simulink model "bldc_DTC_final"  (R2024b)
settings: Solver=VariableStepAuto  StartTime=0.0  StopTime=13  RelTol=1e-3
model workspace (MAT data in the model file):
  Ls = 0.0027
  Rs = 0.7
libraries: spsIGBTDiodeLib x6, spsVoltageMeasurementLib x3, simulink x2, spsPermanentMagnetSynchronousMachineLib x1, spsDCVoltageSourceLib x1, simulink_extras x1, slpidlib x1, spsThreePhaseVIMeasurementLib x1, spspowerguiLib x1
settings Model: Creator=INNAGOL2  LastModifiedBy=INNAGOL2

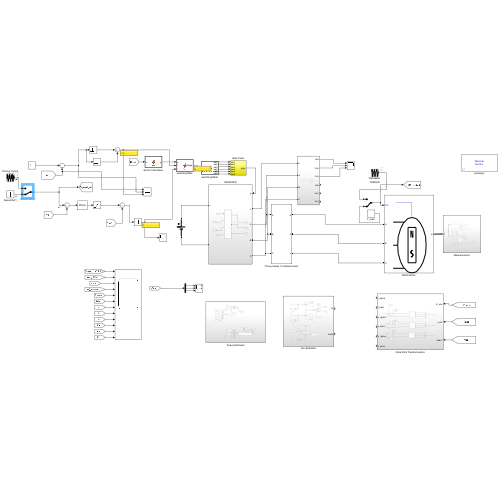
[thumbnail: Simulink's stored preview of the top-level diagram]
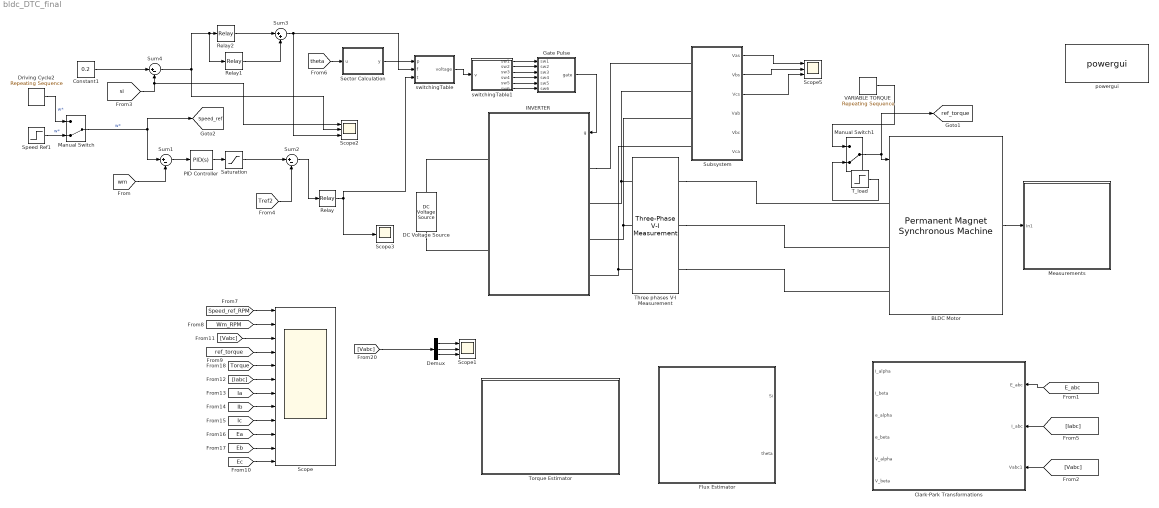
== system bldc_DTC_final ==
  BLDC Motor : spsPermanentMagnetSynchronousMachineLib/Permanent Magnet Synchronous Machine  NbPhases=3  FluxDistribution=Trapezoidal  RotorType=Round  MechanicalLoad=Torque Tm  PresetModel=No  ShowDetailedParameters=on  MeasurementBus=off  Resistance=0.7  Inductance=2.7e-3  dqInductances=[8.5e-3,8.5e-3]  La=0.000835  MachineConstant=Flux linkage established by magnets (V.s)  Flux=0.1194  VoltageCst=100.0283  TorqueCst=0.9552  Flat=120  Mechanical=[0.0027 0.0004924 4]  PolePairs=4  InitialConditions=[0,0, 0,0]  InitialConditions5ph=[0 0 0 0 0 0]  RefAngle=Aligned with phase A axis (original Park)  IterativeDiscreteModel=Trapezoidal non iterative  TsBlock=-1  TsPowergui=0
  Clark-Park Transformations : Subsystem
  Constant1 : Constant  Value=0.2
  DC Voltage Source : spsDCVoltageSourceLib/DC Voltage Source  Amplitude=160  Measurements=None
  Demux : Demux  Outputs=3
  Driving Cycle2 : simulink/Sources/Repeating Sequence  rep_seq_t=[0 1 2 3 4 5 6 7 8 9 10 11 11.0001 12 13]  rep_seq_y=[0 200 200 0 0 0 -100 -100 0 0 150 150 140 140 0]
  Flux Estimator : Subsystem
  Gate Pulse : Subsystem
  INVERTER : Subsystem
  Manual Switch : ManualSwitch  CurrentSetting=0
  Manual Switch1 : ManualSwitch  CurrentSetting=0
  Measurements : Subsystem
  PID Controller : slpidlib/PID Controller  Controller=PID  Form=Parallel  TimeDomain=Continuous-time  UseExternalTs=off  SampleTime=-1  IntegratorMethod=Forward Euler  FilterMethod=Forward Euler  ControllerParametersSource=internal  P=18  I=35  UseKiTs=off  D=0  UseExternalDerivativeSource=off  N=100  UseFilter=on  TunerSelectOption=Transfer Function Based (PID Tuner App)  InitialConditionSource=internal  InitialConditionForIntegrator=0  InitialConditionForFilter=0  DifferentiatorICPrevScaledInput=0  ExternalReset=none  TrackingMode=off  Kt=1  LimitOutput=off  SatLimitsSource=internal  UpperSaturationLimit=inf  LowerSaturationLimit=-inf  LinearizeAsGain=on  AntiWindupMode=none  Kb=1  LimitIntegrator=off  UpperIntegratorSaturationLimit=inf  LowerIntegratorSaturationLimit=-inf  POutMin=[]  POutMax=[]  IOutMin=[]  IOutMax=[]  DOutMin=[]  DOutMax=[]  NOutMin=[]  NOutMax=[]  SumOutMin=[]  SumOutMax=[]  SaturationOutMin=[]  SaturationOutMax=[]  PParamMin=[]  PParamMax=[]  IParamMin=[]  IParamMax=[]  DParamMin=[]  DParamMax=[]  NParamMin=[]  NParamMax=[]  KbParamMin=[]  KbParamMax=[]  KtParamMin=[]  KtParamMax=[]  KbOutMin=[]  KbOutMax=[]  KtOutMin=[]  KtOutMax=[]  IntegratorOutMin=[]  IntegratorOutMax=[]  FilterOutMin=[]  FilterOutMax=[]  SumI1OutMin=[]  SumI1OutMax=[]  SumI2OutMin=[]  SumI2OutMax=[]  SumI3OutMin=[]  SumI3OutMax=[]  SumI4OutMin=[]  SumI4OutMax=[]  SumDOutMin=[]  SumDOutMax=[]  DifferentiatorOutMin=[]  DifferentiatorOutMax=[]  FilterDiffOutCoefMin=[]  FilterDiffOutCoefMax=[]  ReciprocalOutMin=[]  ReciprocalOutMax=[]  SumDenOutMin=[]  SumDenOutMax=[]  SumNumOutMin=[]  SumNumOutMax=[]  DivideOutMin=[]  DivideOutMax=[]  UdiffTsProdOutMin=[]  UdiffTsProdOutMax=[]  NTsProdOutMin=[]  NTsProdOutMax=[]  UintegralTsProdOutMin=[]  UintegralTsProdOutMax=[]  UngainTsProdOutMin=[]  UngainTsProdOutMax=[]  ClampingZeroOutDataTypeStr=Inherit: Inherit via back propagation  ClampingZeroOutMin=[]  ClampingZeroOutMax=[]  FilterDenConstantOutDataTypeStr=Inherit: Inherit via back propagation  FilterDenConstantOutMin=[]  FilterDenConstantOutMax=[]  PCopyOutDataTypeStr=Inherit: Inherit via back propagation  PCopyOutMin=[]  PCopyOutMax=[]  NCopyOutDataTypeStr=Inherit: Inherit via back propagation  NCopyOutMin=[]  NCopyOutMax=[]  IntegratorContinuousStateAttributes=''  IntegratorStateMustResolveToSignalObject=off  IntegratorRTWStateStorageClass=Auto  FilterContinuousStateAttributes=''  FilterStateMustResolveToSignalObject=off  FilterRTWStateStorageClass=Auto  ParallelPVariant=InternalParameters  IdealPVariant=Disabled  IVariant=InternalParameters  DVariant=InternalParameters  IntegratorVariant=Continuous  SatVariant=Disabled  AWVariant=Passthrough  PCopyVariant=Disabled  TRVariant=Disabled  FdbkBlocksVariant=Forward  IdealPFdbkVariant=Disabled  SatFdbkVariant=Disabled  DerivativeFilterVariant=ContFilter  NVariant=InternalParameters  NCopyVariant=Disabled  FilterICVariant=InternalICsFilter  IntegratorICVariant=InternalICs  ExternalResetVariant=Disabled  TRSumVariant=Passthrough  SumFdbkVariant=Disabled  SumVariant=Sum_PID  TsampFilterVariant=InternalTs  TsampNgainVariant=Passthrough  TsampIntegralVariant=Disabled_SignalSpec  ExternalSaturationOutDataTypeStr=Inherit: Same as second input  DerivativeSourceVariant=ErrorSignal  PreIntVariant=InternalPreInt
  Relay : Relay  OnSwitchValue=1  OffSwitchValue=0  OnOutputValue=1  OffOutputValue=-1
  Relay1 : Relay  OnSwitchValue=0  OffSwitchValue=-0.01  OnOutputValue=0  OffOutputValue=-1
  Relay2 : Relay  OnSwitchValue=0.01  OffSwitchValue=0
  Saturation : Saturate  UpperLimit=25  LowerLimit=-25
  Scope : Scope  NumInputPorts=12
  Scope1 : Scope  NumInputPorts=3
  Scope2 : Scope  NumInputPorts=3
  Scope3 : Scope
  Scope5 : Scope  NumInputPorts=3
  Sector Calculation : MATLAB Function  TreatAsAtomicUnit=on
  Speed Ref1 : Step  Time=0.1  After=-150  SampleTime=0
  Subsystem : Subsystem
  Sum1 : Sum  Inputs=|+-
  Sum2 : Sum  Inputs=|+-
  Sum3 : Sum  Inputs=|++
  Sum4 : Sum  Inputs=|+-
  "T_load " : Step  Time=0.1  After=5  SampleTime=0
  Three phases V-I Measurement : spsThreePhaseVIMeasurementLib/Three-Phase V-I Measurement  VoltageMeasurement=phase-to-phase  SetLabelV=on  LabelV=Vabc  Vpu=off  VpuLL=off  CurrentMeasurement=yes  SetLabelI=on  LabelI=Iabc  Ipu=off  Pbase=100e6  Vbase=500e3  OutputType=Complex  PhasorSimulation=off  PSBequivalent=0
  Torque Estimator : Subsystem
  VARIABLE TORQUE : simulink/Sources/Repeating Sequence  rep_seq_t=[0 1 2 3 4 5 6 7 8 9 10 11 12 13]  rep_seq_y=[3 3 3 3 5 5 5 -2 -2 -2 1 1 1 1 ]
  powergui : spspowerguiLib/powergui  Priority=1  SimulationMode=Discrete  SampleTime=5e-05  frequency=60  Iterations=50  frequencyindice=0  Pbase=100e6  ErrMax=1e-4  UnitsV=kV  UnitsW=MW  buscounter=0  FunctionMessages=off  echomessages=off  EnableUseOfTLC=off  CurrentSourceSwitches=off  DisableSnubberDevices=off  DisableRonSwitches=off  DisableVfSwitches=off  DisplayEquations=off  AutomaticDiscreteSolvers=off  SolverType=Tustin/Backward Euler (TBE)  Interpol=off  ExternalGateDelay=off  methode=off  Ts=100  x0status=blocks  SPID=on  SwTol=0  HookPort=off  NonlinearTolerance=1e-4  nMaxIteration=100  ContinueOnMaxIteration=off  RestoreLinks=warning  ResistiveCurrentMeasurement=off  Frange=[0:2:500]  Ylog=off  Xlog=on  ShowGrid=off  save=off  variable=ZData  structure=0  ZoomFFT=off  StartTime=0.0  cycles=1  DisplayStyle=1  fundamental=60  FreqAxis=off  MaxFrequency=1000  frequencyindicesteady=1  RmsSteady=1  display=off
  switchingTable : MATLAB Function  TreatAsAtomicUnit=on
  switchingTable1 : MATLAB Function  TreatAsAtomicUnit=on
  tag scope: Speed_ref=global, ref_torque=global
  wires:
  PID Controller/1 -> Saturation/1
  Sum1/1 -> PID Controller/1
  Constant1/1 -> Sum4/1
  [wm] -> Sum1/2
  Saturation/1 -> Sum2/1
  VARIABLE TORQUE/1 -> Manual Switch1/1
  Manual Switch1/1 -> BLDC Motor/1, [ref_torque]
  Gate Pulse/1(gate) -> INVERTER/1(g)
  BLDC Motor/1 -> Measurements/1(In1)
  "T_load "/1 -> Manual Switch1/2
  [Iabc] -> Clark-Park Transformations/2(I_abc)
  [E_abc] -> Clark-Park Transformations/1(E_abc)
  [Vabc] -> Clark-Park Transformations/3(Vabc1)
  Manual Switch/1 -> Sum1/1, [Speed_ref]  "w*"
  Sum2/1 -> Relay/1
  Sum4/1 -> Scope2/2, Relay1/1, Relay2/1
  [si] -> Scope2/1, Sum4/2
  [Tref2] -> Sum2/2
  Sector Calculation/1(y) -> switchingTable/1(p)
  [theta] -> Sector Calculation/1(u)
  [Ic] -> Scope/9
  [Ec] -> Scope/12
  [Ea] -> Scope/10
  [Eb] -> Scope/11
  [Vabc] -> Scope/3
  [Torque] -> Scope/5
  [Wm_RPM] -> Scope/2
  [Iabc] -> Scope/6
  [Ib] -> Scope/8
  [Ia] -> Scope/7
  [ref_torque] -> Scope/4
  [Speed_ref_RPM] -> Scope/1
  Driving Cycle2/1 -> Manual Switch/1  "w*"
  Speed Ref1/1 -> Manual Switch/2  "w*"
  [Vabc] -> Demux/1
  Demux/1 -> Scope1/1
  Demux/2 -> Scope1/2
  Demux/3 -> Scope1/3
  Relay/1 -> Scope3/1, switchingTable/3(t)
  switchingTable1/1(sw1) -> Gate Pulse/1(sw1)
  switchingTable1/2(sw2) -> Gate Pulse/2(sw2)
  switchingTable1/3(sw3) -> Gate Pulse/3(sw3)
  switchingTable1/4(sw4) -> Gate Pulse/4(sw4)
  switchingTable1/5(sw5) -> Gate Pulse/5(sw5)
  switchingTable1/6(sw6) -> Gate Pulse/6(sw6)
  switchingTable/1(voltage) -> switchingTable1/1(v)
  Relay2/1 -> Sum3/1
  Relay1/1 -> Sum3/2
  Sum3/1 -> Scope2/3, switchingTable/2(f)
  Subsystem/1(Vas) -> Scope5/1
  Subsystem/2(Vbs) -> Scope5/2
  Subsystem/3(Vcs) -> Scope5/3
  connections:
  Three phases V-I Measurement/LConn3 -- Subsystem/LConn4 -- INVERTER/LConn4
  DC Voltage Source/RConn1 -- INVERTER/RConn1
  Three phases V-I Measurement/LConn2 -- INVERTER/LConn3 -- Subsystem/LConn3
  DC Voltage Source/LConn1 -- INVERTER/RConn2
  Three phases V-I Measurement/LConn1 -- Subsystem/LConn2 -- INVERTER/LConn2
  INVERTER/LConn1 -- Subsystem/LConn1
  Three phases V-I Measurement/RConn1 -- BLDC Motor/LConn1
  Three phases V-I Measurement/RConn2 -- BLDC Motor/LConn2
  Three phases V-I Measurement/RConn3 -- BLDC Motor/LConn3

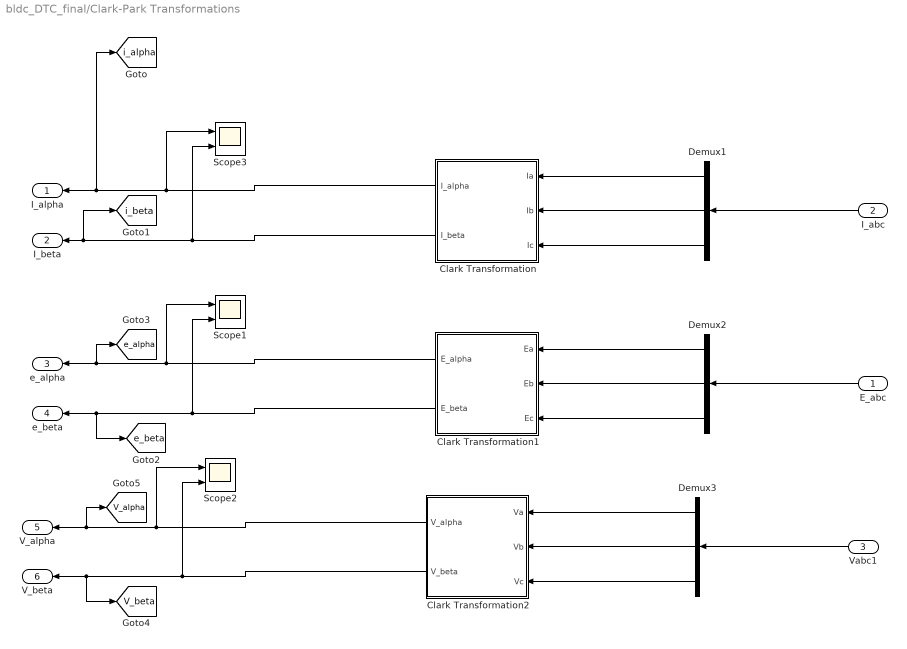
== system bldc_DTC_final/Clark-Park Transformations ==
  E_abc : Inport
  I_abc : Inport  Port=2
  Vabc1 : Inport  Port=3
  Clark Transformation : Subsystem
  Clark Transformation1 : Subsystem
  Clark Transformation2 : Subsystem
  Demux1 : Demux  Outputs=3
  Demux2 : Demux  Outputs=3
  Demux3 : Demux  Outputs=3
  Scope1 : Scope  NumInputPorts=2
  Scope2 : Scope  NumInputPorts=2
  Scope3 : Scope  NumInputPorts=2
  I_alpha : Outport
  I_beta : Outport  Port=2
  e_alpha : Outport  Port=3
  e_beta : Outport  Port=4
  V_alpha : Outport  Port=5
  V_beta : Outport  Port=6
  tag scope: V_alpha=global, V_beta=global, e_alpha=global, e_beta=global, i_alpha=global, i_beta=global
  wires:
  Demux1/1 -> Clark Transformation/1(Ia)
  Demux1/2 -> Clark Transformation/2(Ib)
  Demux1/3 -> Clark Transformation/3(Ic)
  I_abc/1 -> Demux1/1
  Clark Transformation/1(I_alpha) -> Scope3/1, [i_alpha], I_alpha/1
  Clark Transformation/2(I_beta) -> Scope3/2, [i_beta], I_beta/1
  Clark Transformation1/2(E_beta) -> [e_beta], e_beta/1, Scope1/2
  Clark Transformation1/1(E_alpha) -> [e_alpha], e_alpha/1, Scope1/1
  E_abc/1 -> Demux2/1
  Demux2/3 -> Clark Transformation1/3(Ec)
  Demux2/2 -> Clark Transformation1/2(Eb)
  Demux2/1 -> Clark Transformation1/1(Ea)
  Demux3/1 -> Clark Transformation2/1(Va)
  Demux3/2 -> Clark Transformation2/2(Vb)
  Demux3/3 -> Clark Transformation2/3(Vc)
  Vabc1/1 -> Demux3/1
  Clark Transformation2/1(V_alpha) -> Scope2/1, V_alpha/1, [V_alpha]
  Clark Transformation2/2(V_beta) -> Scope2/2, V_beta/1, [V_beta]

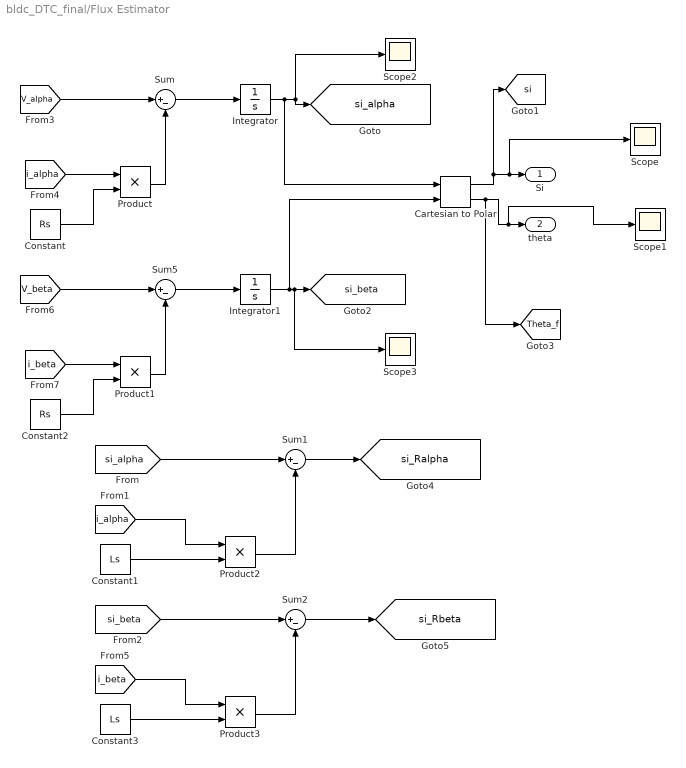
== system bldc_DTC_final/Flux Estimator ==
  Cartesian to Polar : simulink_extras/Transformations/Cartesian to Polar
  Constant : Constant  Value=Rs
  Constant1 : Constant  Value=Ls
  Constant2 : Constant  Value=Rs
  Constant3 : Constant  Value=Ls
  Integrator : Integrator
  Integrator1 : Integrator
  Product{,1..3} (4 alike) : Product
  Scope{,1..3} (4 alike) : Scope
  Sum{,1..2,5} (4 alike) : Sum  Inputs=|+-
  Si : Outport
  theta : Outport  Port=2
  tag scope: Theta_f=global, si=global, si_Ralpha=global, si_Rbeta=global, si_alpha=global, si_beta=global
  wires:
  Constant/1 -> Product/2
  Integrator/1 -> Cartesian to Polar/1, Scope2/1, [si_alpha]
  [V_alpha] -> Sum/1
  [i_alpha] -> Product/1
  Product1/1 -> Sum5/2
  Product/1 -> Sum/2
  [i_beta] -> Product1/1
  Constant2/1 -> Product1/2
  Sum5/1 -> Integrator1/1
  [V_beta] -> Sum5/1
  Integrator1/1 -> Cartesian to Polar/2, Scope3/1, [si_beta]
  Sum/1 -> Integrator/1
  Cartesian to Polar/1 -> [si], Scope/1, Si/1
  Cartesian to Polar/2 -> [Theta_f], Scope1/1, theta/1
  [si_alpha] -> Sum1/1
  [i_alpha] -> Product2/1
  Constant1/1 -> Product2/2
  Product2/1 -> Sum1/2
  Product3/1 -> Sum2/2
  Constant3/1 -> Product3/2
  [i_beta] -> Product3/1
  [si_beta] -> Sum2/1
  Sum1/1 -> [si_Ralpha]
  Sum2/1 -> [si_Rbeta]

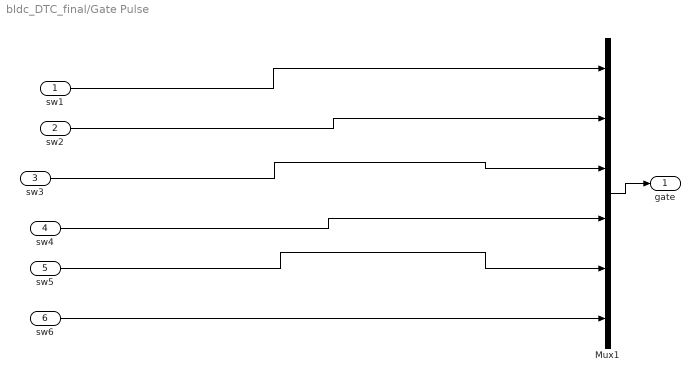
== system bldc_DTC_final/Gate Pulse ==
  sw1 : Inport
  sw2 : Inport  Port=2
  sw3 : Inport  Port=3
  sw4 : Inport  Port=4
  sw5 : Inport  Port=5
  sw6 : Inport  Port=6
  Mux1 : Mux  Inputs=6
  gate : Outport
  wires:
  sw5/1 -> Mux1/5
  Mux1/1 -> gate/1
  sw3/1 -> Mux1/3
  sw1/1 -> Mux1/1
  sw2/1 -> Mux1/2
  sw4/1 -> Mux1/4
  sw6/1 -> Mux1/6

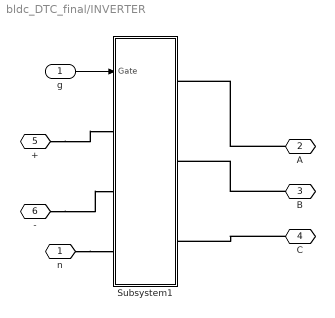
== system bldc_DTC_final/INVERTER ==
  g : Inport
  Subsystem1 : Subsystem
  " n" : PMIOPort  Side=Left
  A : PMIOPort  Port=2  Side=Left
  B : PMIOPort  Port=3  Side=Left
  C : PMIOPort  Port=4  Side=Left
  + : PMIOPort  Port=5  Side=Right
  - : PMIOPort  Port=6  Side=Right
  wires:
  g/1 -> Subsystem1/1(Gate)
  connections:
  +/RConn1 -- Subsystem1/LConn1
  -/RConn1 -- Subsystem1/LConn2
  C/RConn1 -- Subsystem1/RConn3
  B/RConn1 -- Subsystem1/RConn2
  A/RConn1 -- Subsystem1/RConn1
  " n"/RConn1 -- Subsystem1/LConn3

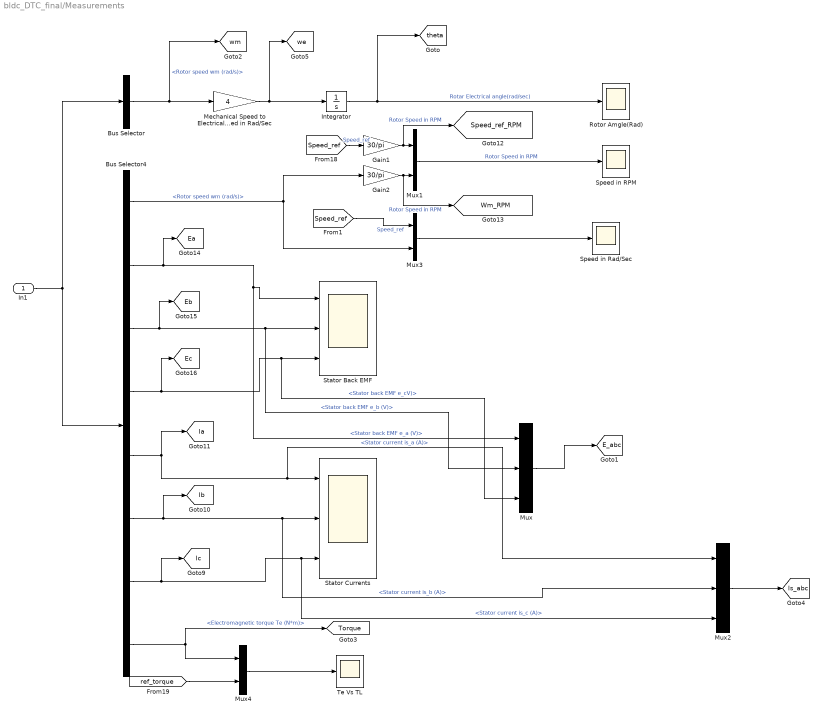
== system bldc_DTC_final/Measurements ==
  In1 : Inport
  Bus Selector : BusSelector  OutputSignals=Rotor speed wm (rad/s)
  Bus Selector4 : BusSelector  OutputSignals=Rotor speed wm (rad/s),Stator back EMF e_a (V),Stator back EMF e_b (V),Stator back EMF e_cV),Stator current is_a (A),Stator current is_b (A),Stator current is_c (A),Electromagnetic torque Te (N*m)
  Gain1 : Gain  Gain=30/pi
  Gain2 : Gain  Gain=30/pi
  Integrator : Integrator  WrapState=on
  Mechanical Speed to Electrical speed in Rad/Sec : Gain  Gain=4
  Mux : Mux  Inputs=3
  Mux1 : Mux  Inputs=2
  Mux2 : Mux  Inputs=3
  Mux3 : Mux  Inputs=2
  Mux4 : Mux  Inputs=2
  Rotor Amgle(Rad) : Scope
  Speed in RPM : Scope
  Speed in Rad/Sec : Scope
  Stator Back EMF : Scope  NumInputPorts=3
  Stator Currents : Scope  NumInputPorts=3
  Te Vs TL : Scope
  tag scope: E_abc=global, Ea=global, Eb=global, Ec=global, Ia=global, Ib=global, Ic=global, Is_abc=global, Speed_ref_RPM=global, Torque=global, Wm_RPM=global, theta=global, we=global, wm=global
  wires:
  [ref_torque] -> Mux4/2
  Mechanical Speed to Electrical speed in Rad/Sec/1 -> [we], Integrator/1
  Mux4/1 -> Te Vs TL/1
  Bus Selector/1 -> [wm], Mechanical Speed to Electrical speed in Rad/Sec/1  "<Rotor speed wm (rad/s)>"
  Bus Selector4/3 -> [Eb], Mux/2, Stator Back EMF/2  "<Stator back EMF e_b (V)>"
  Bus Selector4/8 -> [Torque], Mux4/1  "<Electromagnetic torque Te (N*m)>"
  Bus Selector4/5 -> [Ia], Mux2/1, Stator Currents/1  "<Stator current is_a (A)>"
  In1/1 -> Bus Selector4/1, Bus Selector/1
  Bus Selector4/4 -> [Ec], Mux/3, Stator Back EMF/3  "<Stator back EMF e_cV)>"
  Gain2/1 -> [Wm_RPM], Mux1/2  "Rotor Speed in RPM"
  Bus Selector4/7 -> [Ic], Mux2/3, Stator Currents/3  "<Stator current is_c (A)>"
  Integrator/1 -> [theta], Rotor Amgle(Rad)/1  "Rotar Electrical angle(rad/sec)"
  Bus Selector4/2 -> [Ea], Mux/1, Stator Back EMF/1  "<Stator back EMF e_a (V)>"
  Bus Selector4/1 -> Mux3/2, Gain2/1  "<Rotor speed wm (rad/s)>"
  Gain1/1 -> [Speed_ref_RPM], Mux1/1  "Rotor Speed in RPM"
  Mux3/1 -> Speed in Rad/Sec/1
  Mux1/1 -> Speed in RPM/1  "Rotor Speed in RPM"
  [Speed_ref] -> Gain1/1  "Speed_ref"
  Bus Selector4/6 -> [Ib], Mux2/2, Stator Currents/2  "<Stator current is_b (A)>"
  [Speed_ref] -> Mux3/1  "Speed_ref"
  Mux/1 -> [E_abc]
  Mux2/1 -> [Is_abc]

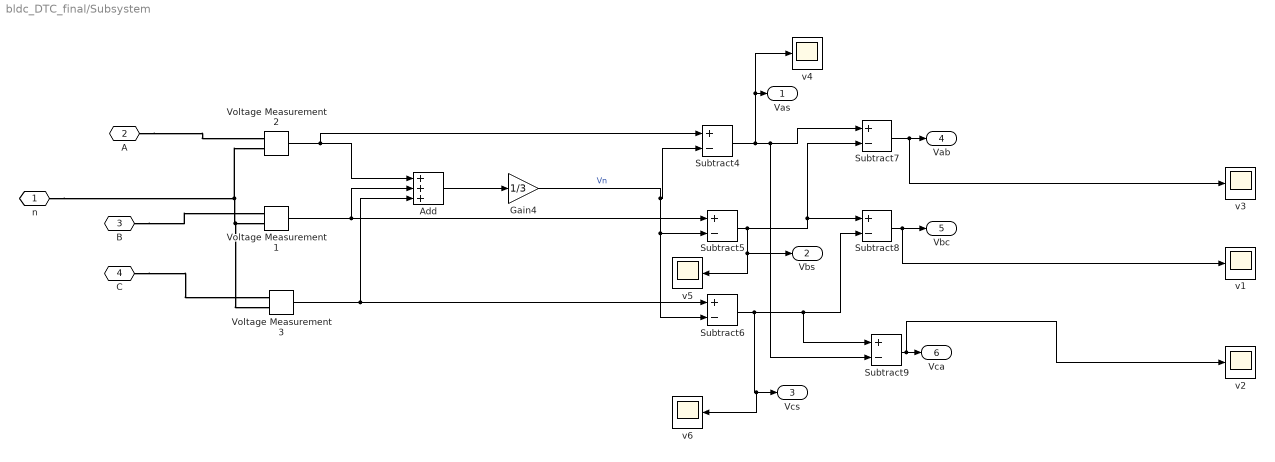
== system bldc_DTC_final/Subsystem ==
  Add : Sum  Inputs=+++
  Gain4 : Gain  Gain=1/3
  Subtract{4..9} (6 alike) : Sum  Inputs=+-
  Voltage Measurement1 : spsVoltageMeasurementLib/Voltage Measurement  PhasorSimulation=off  OutputType=Complex  PSBequivalent=0
  Voltage Measurement2 : spsVoltageMeasurementLib/Voltage Measurement  PhasorSimulation=off  OutputType=Complex  PSBequivalent=0
  Voltage Measurement3 : spsVoltageMeasurementLib/Voltage Measurement  PhasorSimulation=off  OutputType=Complex  PSBequivalent=0
  v{1..6} (6 alike) : Scope
  n : PMIOPort  Side=Left
  A : PMIOPort  Port=2  Side=Left
  B : PMIOPort  Port=3  Side=Left
  C : PMIOPort  Port=4  Side=Left
  Vas : Outport  VectorParamsAs1DForOutWhenUnconnected=off
  Vbs : Outport  Port=2  VectorParamsAs1DForOutWhenUnconnected=off
  Vcs : Outport  Port=3  VectorParamsAs1DForOutWhenUnconnected=off
  Vab : Outport  Port=4  VectorParamsAs1DForOutWhenUnconnected=off
  Vbc : Outport  Port=5  VectorParamsAs1DForOutWhenUnconnected=off
  Vca : Outport  Port=6  VectorParamsAs1DForOutWhenUnconnected=off
  wires:
  Voltage Measurement2/1 -> Subtract4/1, Add/1
  Voltage Measurement1/1 -> Subtract5/1, Add/2
  Voltage Measurement3/1 -> Subtract6/1, Add/3
  Add/1 -> Gain4/1
  Subtract4/1 -> v4/1, Vas/1, Subtract9/2, Subtract7/1
  Subtract5/1 -> v5/1, Vbs/1, Subtract8/1, Subtract7/2
  Subtract6/1 -> v6/1, Vcs/1, Subtract9/1, Subtract8/2
  Subtract7/1 -> v3/1, Vab/1
  Subtract8/1 -> v1/1, Vbc/1
  Subtract9/1 -> v2/1, Vca/1
  Gain4/1 -> Subtract6/2, Subtract5/2, Subtract4/2  "Vn"
  connections:
  n/RConn1 -- Voltage Measurement2/LConn2 -- Voltage Measurement3/LConn2 -- Voltage Measurement1/LConn2
  A/RConn1 -- Voltage Measurement2/LConn1
  B/RConn1 -- Voltage Measurement1/LConn1
  C/RConn1 -- Voltage Measurement3/LConn1

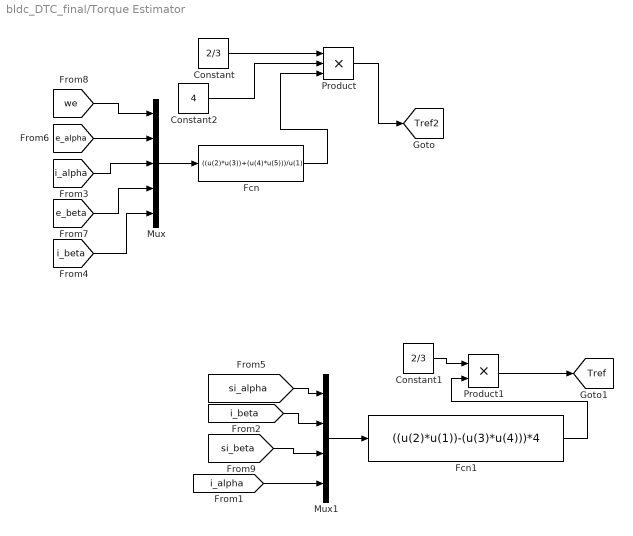
== system bldc_DTC_final/Torque Estimator ==
  Constant : Constant  Value=2/3
  Constant1 : Constant  Value=2/3
  Constant2 : Constant  Value=4
  Fcn : Fcn  Expr=((u(2)*u(3))+(u(4)*u(5)))/u(1)
  Fcn1 : Fcn  Expr=((u(2)*u(1))-(u(3)*u(4)))*4
  Mux : Mux  Inputs=5
  Mux1 : Mux
  Product : Product  Inputs=3
  Product1 : Product
  tag scope: Tref2=global, Tref=global
  wires:
  Constant/1 -> Product/1
  [i_beta] -> Mux/5
  [i_alpha] -> Mux/3
  Mux/1 -> Fcn/1
  Product/1 -> [Tref2]
  [e_beta] -> Mux/4
  Fcn/1 -> Product/3
  [we] -> Mux/1
  [e_alpha] -> Mux/2
  Constant2/1 -> Product/2
  [si_beta] -> Mux1/3
  [si_alpha] -> Mux1/1
  Mux1/1 -> Fcn1/1
  [i_beta] -> Mux1/2
  [i_alpha] -> Mux1/4
  Product1/1 -> [Tref]
  Constant1/1 -> Product1/1
  Fcn1/1 -> Product1/2

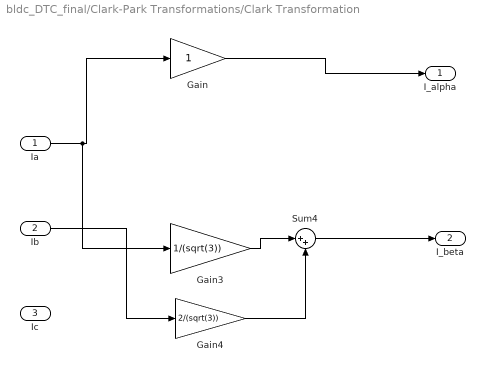
== system bldc_DTC_final/Clark-Park Transformations/Clark Transformation ==
  Ia : Inport
  Ib : Inport  Port=2
  Ic : Inport  Port=3
  Gain : Gain
  Gain3 : Gain  Gain=1/(sqrt(3))
  Gain4 : Gain  Gain=2/(sqrt(3))
  Sum4 : Sum  Inputs=|++
  I_alpha : Outport
  I_beta : Outport  Port=2
  wires:
  Gain/1 -> I_alpha/1
  Gain3/1 -> Sum4/1
  Gain4/1 -> Sum4/2
  Ia/1 -> Gain3/1, Gain/1
  Sum4/1 -> I_beta/1
  Ib/1 -> Gain4/1

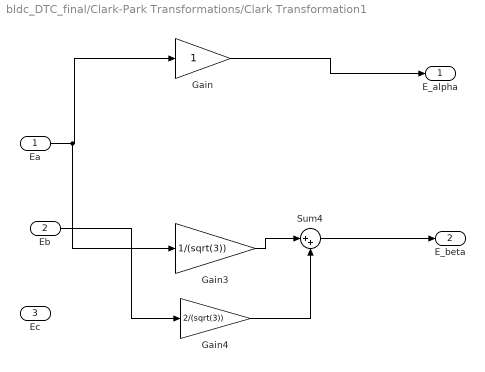
== system bldc_DTC_final/Clark-Park Transformations/Clark Transformation1 ==
  Ea : Inport
  Eb : Inport  Port=2
  Ec : Inport  Port=3
  Gain : Gain
  Gain3 : Gain  Gain=1/(sqrt(3))
  Gain4 : Gain  Gain=2/(sqrt(3))
  Sum4 : Sum  Inputs=|++
  E_alpha : Outport
  E_beta : Outport  Port=2
  wires:
  Gain/1 -> E_alpha/1
  Ea/1 -> Gain3/1, Gain/1
  Eb/1 -> Gain4/1
  Gain3/1 -> Sum4/1
  Sum4/1 -> E_beta/1
  Gain4/1 -> Sum4/2

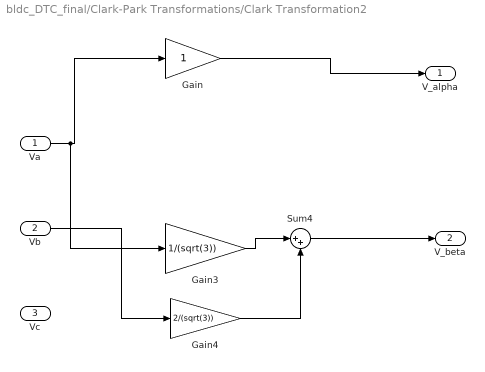
== system bldc_DTC_final/Clark-Park Transformations/Clark Transformation2 ==
  Va : Inport
  Vb : Inport  Port=2
  Vc : Inport  Port=3
  Gain : Gain
  Gain3 : Gain  Gain=1/(sqrt(3))
  Gain4 : Gain  Gain=2/(sqrt(3))
  Sum4 : Sum  Inputs=|++
  V_alpha : Outport
  V_beta : Outport  Port=2
  wires:
  Gain/1 -> V_alpha/1
  Va/1 -> Gain3/1, Gain/1
  Vb/1 -> Gain4/1
  Gain3/1 -> Sum4/1
  Sum4/1 -> V_beta/1
  Gain4/1 -> Sum4/2

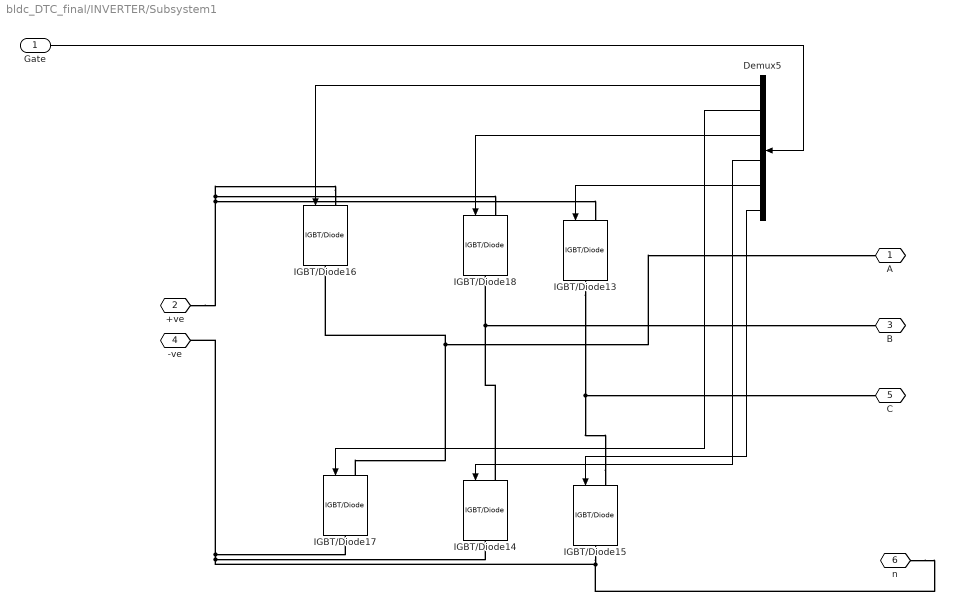
== system bldc_DTC_final/INVERTER/Subsystem1 ==
  Gate : Inport
  Demux5 : Demux  Outputs=6
  IGBT/Diode{13..18} (6 alike) : spsIGBTDiodeLib/IGBT//Diode  Ron=1e-3  Rs=1e5  Cs=inf  Measurements=off
  A : PMIOPort  Side=Right
  +ve : PMIOPort  Port=2  Side=Left
  B : PMIOPort  Port=3  Side=Right
  -ve : PMIOPort  Port=4  Side=Left
  C : PMIOPort  Port=5  Side=Right
  " n" : PMIOPort  Port=6  Side=Left
  wires:
  Gate/1 -> Demux5/1
  Demux5/1 -> IGBT/Diode16/1
  Demux5/2 -> IGBT/Diode17/1
  Demux5/3 -> IGBT/Diode18/1
  Demux5/4 -> IGBT/Diode14/1
  Demux5/5 -> IGBT/Diode13/1
  Demux5/6 -> IGBT/Diode15/1
  connections:
  IGBT/Diode15/LConn1 -- C/RConn1 -- IGBT/Diode13/RConn1
  IGBT/Diode18/RConn1 -- B/RConn1 -- IGBT/Diode14/LConn1
  IGBT/Diode14/RConn1 -- " n"/RConn1 -- IGBT/Diode15/RConn1 -- IGBT/Diode17/RConn1 -- -ve/RConn1
  IGBT/Diode16/RConn1 -- A/RConn1 -- IGBT/Diode17/LConn1
  IGBT/Diode16/LConn1 -- IGBT/Diode18/LConn1 -- +ve/RConn1 -- IGBT/Diode13/LConn1

== matlab function bldc_DTC_final/switchingTable ==
  data: p input; voltage output; f input; t input
function voltage = fcn(p, f, t)
    % Ensure inputs are doubles
    p = double(p);
    f = double(f);
    t = double(t);
    
    % Define the output as a scalar
    voltage = 0; % default value

    % Check if the inputs are valid (scalars)
    if numel(p) ~= 1 || numel(f) ~= 1 || numel(t) ~= 1
        error('Inputs p, f, and t must be scalars');
    end
    
    % Define the logic based on the voltage value of p
    if p == 1
        if f == 1 && t == 1
            voltage = 1;
        elseif f == 0 && t == 1
            voltage = 2;    
        elseif f == -1 && t == 1
            voltage = 3;
        elseif f == 1 && t == 0
            voltage = 1;
        elseif f == 0 && t == 0
            voltage = 0;   
        elseif f == -1 && t == 0
            voltage = 3;
        elseif f == 1 && t == -1
            voltage = 6;
        elseif f == 0 && t == -1
            voltage = 5;   
        elseif f == -1 && t == -1
            voltage = 4;
        end
    elseif p == 2
        if f == 1 && t == 1
            voltage = 2;
        elseif f == 0 && t == 1
            voltage = 3;    
        elseif f == -1 && t == 1
            voltage = 4;
         elseif f == 1 && t == 0
            voltage = 2;
        elseif f == 0 && t == 0
            voltage = 0;   
        elseif f == -1 && t == 0
            voltage = 4;
         elseif f == 1 && t == -1
            voltage = 1;
        elseif f == 0 && t == -1
            voltage = 6;   
        elseif f == -1 && t == -1
            voltage = 5;
        end
    elseif p == 3
        if f == 1 && t == 1
            voltage = 3;
        elseif f == 0 && t == 1
            voltage = 4;    
        elseif f == -1 && t == 1
            voltage = 5;
        elseif f == 1 && t == 0
            voltage = 3;
        elseif f == 0 && t == 0
            voltage = 0;   
        elseif f == -1 && t == 0
            voltage = 5;
        elseif f == 1 && t == -1
            voltage = 2;
        elseif f == 0 && t == -1
            voltage = 1;   
        elseif f == -1 && t == -1
            voltage = 6;        
        end
    elseif p == 4
        if f == 1 && t == 1
            voltage = 4;
        elseif f == 0 && t == 1
            voltage = 5;    
        elseif f == -1 && t == 1
            voltage = 6;
        elseif f == 1 && t == 0
            voltage = 4;
        elseif f == 0 && t == 0
            voltage = 0;   
        elseif f == -1 && t == 0
            voltage = 6;
        elseif f == 1 && t == -1
            voltage = 3;
        elseif f == 0 && t == -1
            voltage = 2;   
        elseif f == -1 && t == -1
            voltage = 1;
        end
    elseif p == 5
        if f == 1 && t == 1
            voltage = 5;
        elseif f == 0 && t == 1
            voltage = 6;    
        elseif f == -1 && t == 1
            voltage = 1;
        elseif f == 1 && t == 0
            voltage = 5;
        elseif f == 0 && t == 0
            voltage = 0;   
        elseif f == -1 && t == 0
            voltage = 1;
        elseif f == 1 && t == -1
            voltage = 4;
        elseif f == 0 && t == -1
            voltage = 3;   
        elseif f == -1 && t == -1
            voltage = 2;
        end
    elseif p == 6
        if f == 1 && t == 1
            voltage = 6;
        elseif f == 0 && t == 1
            voltage = 1;    
        elseif f == -1 && t == 1
            voltage = 2;
        elseif f == 1 && t == 0
            voltage = 6;
        elseif f == 0 && t == 0
            voltage = 0;   
        elseif f == -1 && t == 0
            voltage = 2;
        elseif f == 1 && t == -1
            voltage = 5;
        elseif f == 0 && t == -1
            voltage = 4;   
        elseif f == -1 && t == -1
            voltage = 3;
        end
    end
end

== matlab function bldc_DTC_final/Sector Calculation ==
  data: u input; y output
function y = fcn(u)
if ( u >- pi/6 && u<=pi / 6 )
y = 1;
elseif ( u > pi/6 && u <= pi / 2)
y = 2;
elseif (u > pi/2 && u<= 5*(pi/6))
y = 3;
elseif (u > - 5*(pi/6) && u<= -pi/2)
y = 5;
elseif ( u > - pi/2 && u<=-pi/6)
y = 6;
else
y = 4;
end

== matlab function bldc_DTC_final/switchingTable1 ==
  data: v input; sw1 output; sw2 output; sw3 output; sw4 output; sw5 output; sw6 output
function [sw1, sw2, sw3, sw4, sw5, sw6] = voltage_vector(v)
    % Initialize all switch outputs to 0
    sw1 = 0; sw2 = 0; sw3 = 0; sw4 = 0; sw5 = 0; sw6 = 0;
 
    % Determine the output based on inputs
    
            if v == 1
                sw1 = 1; sw2 = 0; sw3 = 0; sw4 = 0; sw5 = 0; sw6 = 1;
            elseif v == 2
                sw1 = 0; sw2 = 0; sw3 = 1; sw4 = 0; sw5 = 0; sw6 = 1;
            elseif v == 3
                sw1 = 0; sw2 = 1; sw3 = 1; sw4 = 0; sw5 = 0; sw6 = 0;
            elseif v == 4
                sw1 = 0; sw2 = 1; sw3 = 0; sw4 = 0; sw5 = 1; sw6 = 0;
            elseif v == 5
                sw1 = 0; sw2 = 0; sw3 = 0; sw4 = 1; sw5 = 1; sw6 = 0;
            elseif v == 6
                sw1 = 1; sw2 = 0; sw3 = 0; sw4 = 1; sw5 = 0; sw6 = 0;
            else
                sw1 = 0; sw2 = 0; sw3 = 0; sw4 = 0; sw5 = 0; sw6 = 0;
            end
  
end
